simulink model "testeqom"  (Simulink 7.4)
settings: Solver=ode45  StartTime=0.0  StopTime=10.0  RelTol=1e-3
undefined symbols (not defined in the file or in its folder): g, m
settings Model: Creator=alstit04  LastModifiedBy=alstit04

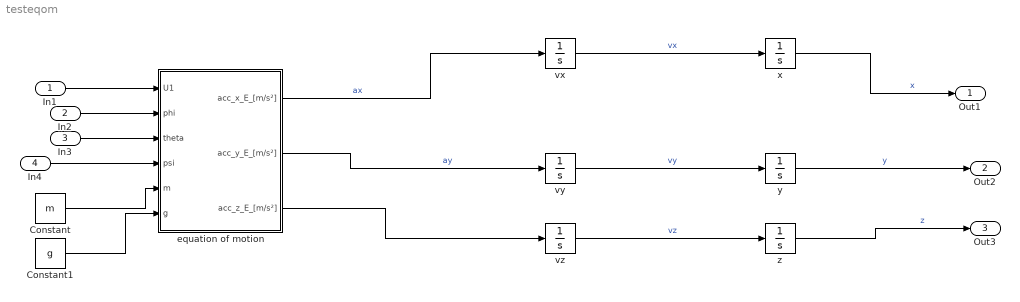
== system testeqom ==
  In1 : Inport  OutDataType=fixdt(1, 16)  OutScaling=2^0
  In2 : Inport  Port=2  OutDataType=fixdt(1, 16)  OutScaling=2^0
  In3 : Inport  Port=3  OutDataType=fixdt(1, 16)  OutScaling=2^0
  In4 : Inport  Port=4  OutDataType=fixdt(1, 16)  OutScaling=2^0
  Constant : Constant  Value=m
  Constant1 : Constant  Value=g
  equation of motion : Subsystem  AncestorBlock=Copter_Library/equation of motion
  vx : Integrator
  vy : Integrator
  vz : Integrator
  x : Integrator
  y : Integrator
  z : Integrator
  Out1 : Outport  OutDataType=fixdt(1, 16)  OutScaling=2^0
  Out2 : Outport  Port=2  OutDataType=fixdt(1, 16)  OutScaling=2^0
  Out3 : Outport  Port=3  OutDataType=fixdt(1, 16)  OutScaling=2^0
  wires:
  vz/1 -> z/1  "vz"
  equation of motion/3(acc_z_E_[m/s²]) -> vz/1
  equation of motion/2(acc_y_E_[m/s²]) -> vy/1  "ay"
  equation of motion/1(acc_x_E_[m/s²]) -> vx/1  "ax"
  In2/1 -> equation of motion/2(phi)
  Constant/1 -> equation of motion/5(m)
  Constant1/1 -> equation of motion/6(g)
  vx/1 -> x/1  "vx"
  vy/1 -> y/1  "vy"
  In3/1 -> equation of motion/3(theta)
  In4/1 -> equation of motion/4(psi)
  In1/1 -> equation of motion/1(U1)
  z/1 -> Out3/1  "z"
  y/1 -> Out2/1  "y"
  x/1 -> Out1/1  "x"

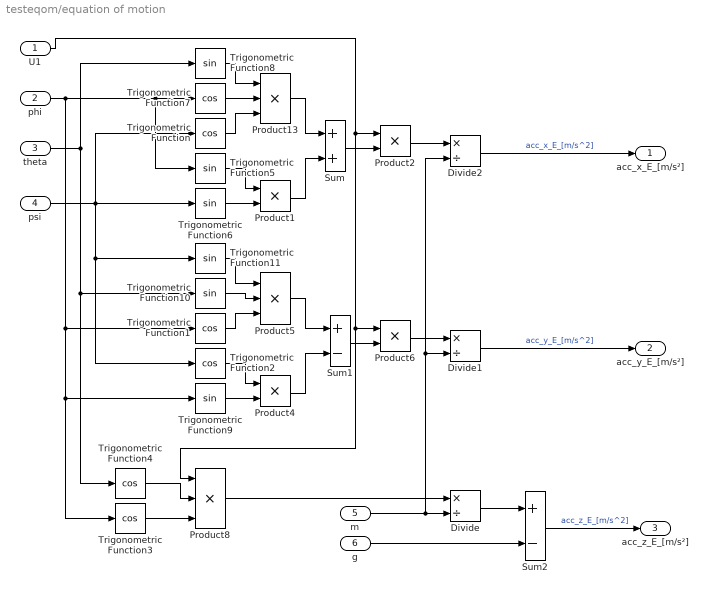
== system testeqom/equation of motion ==
  U1 : Inport  OutDataType=fixdt(1, 16)  OutScaling=2^0
  phi : Inport  Port=2  OutDataType=fixdt(1, 16)  OutScaling=2^0
  theta : Inport  Port=3  OutDataType=fixdt(1, 16)  OutScaling=2^0
  psi : Inport  Port=4  OutDataType=fixdt(1, 16)  OutScaling=2^0
  m : Inport  Port=5  OutDataType=fixdt(1, 16)  OutScaling=2^0
  g : Inport  Port=6  OutDataType=fixdt(1, 16)  OutScaling=2^0
  Divide : Product  Inputs=*/  OutDataType=fixdt(1, 16)  OutScaling=2^-10
  Divide1 : Product  Inputs=*/  OutDataType=fixdt(1, 16)  OutScaling=2^-10
  Divide2 : Product  Inputs=*/  OutDataType=fixdt(1, 16)  OutScaling=2^-10
  Product{1..2,4,6} (4 alike) : Product  OutDataType=fixdt(1, 16)  OutScaling=2^0  RndMeth=Zero
  Product13 : Product  Inputs=3  OutDataType=fixdt(1, 16)  OutScaling=2^0  RndMeth=Zero
  Product5 : Product  Inputs=3  OutDataType=fixdt(1, 16)  OutScaling=2^0  RndMeth=Zero
  Product8 : Product  Inputs=3  OutDataType=fixdt(1, 16)  OutScaling=2^0  RndMeth=Zero
  Sum : Sum  OutDataType=fixdt(1, 16)  OutScaling=2^0
  Sum1 : Sum  Inputs=+-  OutDataType=fixdt(1, 16)  OutScaling=2^0
  Sum2 : Sum  Inputs=+-  OutDataType=fixdt(1, 16)  OutScaling=2^0
  Trigonometric Function{,1..4,7} (6 alike) : Trigonometry  Operator=cos
  Trigonometric Function{5..6,8..11} (6 alike) : Trigonometry
  acc_x_E_[m/s²] : Outport  OutDataType=fixdt(1, 16)  OutScaling=2^0
  acc_y_E_[m/s²] : Outport  Port=2  OutDataType=fixdt(1, 16)  OutScaling=2^0
  acc_z_E_[m/s²] : Outport  Port=3  OutDataType=fixdt(1, 16)  OutScaling=2^0
  wires:
  Sum2/1 -> acc_z_E_[m/s²]/1  "acc_z_E_[m/s^2]"
  m/1 -> Divide2/2, Divide1/2, Divide/2
  U1/1 -> Product2/1, Product6/1, Product8/1
  Product8/1 -> Divide/1
  phi/1 -> Trigonometric Function5/1, Trigonometric Function7/1, Trigonometric Function3/1, Trigonometric Function9/1, Trigonometric Function1/1
  Divide1/1 -> acc_y_E_[m/s²]/1  "acc_y_E_[m/s^2]"
  theta/1 -> Trigonometric Function8/1, Trigonometric Function4/1, Trigonometric Function10/1
  psi/1 -> Trigonometric Function6/1, Trigonometric Function/1, Trigonometric Function11/1, Trigonometric Function2/1
  Trigonometric Function6/1 -> Product1/2
  Trigonometric Function5/1 -> Product1/1
  Product1/1 -> Sum/2
  Trigonometric Function8/1 -> Product13/1
  Trigonometric Function7/1 -> Product13/2
  Trigonometric Function/1 -> Product13/3
  Product13/1 -> Sum/1
  Sum/1 -> Product2/2
  Product2/1 -> Divide2/1
  Trigonometric Function9/1 -> Product4/2
  Trigonometric Function2/1 -> Product4/1
  Product4/1 -> Sum1/2
  Trigonometric Function11/1 -> Product5/1
  Trigonometric Function10/1 -> Product5/2
  Product5/1 -> Sum1/1
  Sum1/1 -> Product6/2
  Product6/1 -> Divide1/1
  Divide2/1 -> acc_x_E_[m/s²]/1  "acc_x_E_[m/s^2]"
  Divide/1 -> Sum2/1
  Trigonometric Function3/1 -> Product8/3
  Trigonometric Function4/1 -> Product8/2
  g/1 -> Sum2/2
  Trigonometric Function1/1 -> Product5/3
